simulink model "Project_2_2020a"  (R2020a)
settings: Solver=ode15s  StartTime=0.0  StopTime=10  MaxStep=0.2  RelTol=1e-2  EnableMultiTasking=on
model workspace (MAT data in the model file):
  g_density = 5
values from neighbouring files (symbols this model uses):
  Aa = 0    [execute_model_2020a.m]
  Ab = 0    [execute_model_2020a.m]
  Ac = 0    [execute_model_2020a.m]
  Ax = 0    [execute_model_2020a.m]
  Ay = 0    [execute_model_2020a.m]
  Az = 0    [execute_model_2020a.m]
  B = [24.233423136094 6.1219332628706 -6.1219332628706 -24.233423136094 -18.111489873223 18.111489873223 ... (first row only)    [execute_model_2020a.m]
  flange_len = 3    [execute_model_2020a.m]
  flange_thick = 0.8    [execute_model_2020a.m]
  flange_width = 2.25    [execute_model_2020a.m]
  hex_skew = -0.25    [execute_model_2020a.m]
  ka = 0    [execute_model_2020a.m]
  kb = 0    [execute_model_2020a.m]
  kc = 0    [execute_model_2020a.m]
  Kd = 8    [execute_model_2020a.m]
  Ki = 11.5    [execute_model_2020a.m]
  Kp = 450    [execute_model_2020a.m]
  kx = 0    [execute_model_2020a.m]
  ky = 0    [execute_model_2020a.m]
  kz = 75    [execute_model_2020a.m]
  leg_rad = 3    [execute_model_2020a.m]
  nom_length = 30    [execute_model_2020a.m]
  P = [14.574164873203 11.040422061358 -11.040422061358 -14.574164873203 -3.5337428118454 3.5337428118454 ... (first row only)    [execute_model_2020a.m]
  pa = 0    [execute_model_2020a.m]
  pb = 0    [execute_model_2020a.m]
  pc = 0    [execute_model_2020a.m]
  platform_rad = 18    [execute_model_2020a.m]
  platform_thick = 2    [execute_model_2020a.m]
  px = 0    [execute_model_2020a.m]
  py = 0    [execute_model_2020a.m]
  pz = 0    [execute_model_2020a.m]
  wa = 0    [execute_model_2020a.m]
  wb = 0    [execute_model_2020a.m]
  wc = 0    [execute_model_2020a.m]
  wx = 0    [execute_model_2020a.m]
  wy = 0    [execute_model_2020a.m]
  wz = 0    [execute_model_2020a.m]
undefined symbols (not defined in the file or in its folder): X, Y, Z
libraries: sm_stewart_platform_lib x13, sm_lib x10, nesl_utility x8, simulink x2, Parts_Lib x1, Contact_Forces_Lib x1, simulink_extras x1
(part 1 of 2)
Description:
  | Stewart Platform
  | 
  | This model shows a Stewart platform manipulator that can track a
  | parameterized reference trajectory. The shape, size, and kinematics of
  | the manipulator are highly configurable.
  | 
  | The reference trajectory is
  | specified in 6-D pose space, and an inverse kinematics module
  | converts it into one through 6-D leg position space.  A generic PID
  | controller attempts to drive the manipulator along the desired
  | trajectory.
settings Model: FPTRunName=Active  Creator=The MathWorks, Inc.  LastModifiedBy=sjain238
settings SolverCC: ZeroCrossAlgorithm=Adaptive
settings DataIOCC: LimitDataPoints=on  SaveFormat=Array  ReturnWorkspaceOutputs=off
settings OptimizationCC: ExpressionDepthLimit=2147483647  LifeSpan=inf
settings DebuggingCC: UnderspecifiedInitializationDetection=Classic  MergeDetectMultiDrivingBlocksExec=none  IgnoredZcDiagnostic=none  SolverPrmCheckMsg=warning  FcnCallInpInsideContextMsg=warning  StateNameClashWarn=warning  SFUnexpectedBacktrackingDiag=warning  SFNoUnconditionalDefaultTransitionDiag=warning  SFExecutionAtInitializationDiag=none  ArithmeticOperatorsInVariantConditions=warning
settings HardwareCC: ProdBitPerPointer=32  ProdBitPerSizeT=32  ProdBitPerPtrDiffT=32  ProdLargestAtomicFloat=None  ProdIntDivRoundTo=Undefined  ProdEndianess=Unspecified  ProdWordSize=32  ProdHWDeviceType=32-bit Generic
settings ModelReferenceCC: PropagateSignalLabelsOutOfModel=off
settings SFSimCC: SimUseLocalCustomCode=off  CustomCodeUndefinedFunction=UseInterfaceOnly
settings RTWCC: RTWUseLocalCustomCode=off
settings CodeAppCC: StateflowObjectComments=on
settings GRTTargetCC: TargetLangStandard=C89/C90 (ANSI)  CombineOutputUpdateFcns=off  GRTInterface=on
settings ConfigComp: CovMetricSettings=dw  CovSaveCumulativeToWorkspaceVar=on  CovSaveSingleToWorkspaceVar=on  CovExternalEMLEnable=off
settings SimscapeCC: SimscapeNormalizeSystem=off  SimscapeLogDataHistory=15000
settings ConfigurationSet: Description=SimMechanics 2G
settings DiagnosticsConfigSet: SimMechanicsRigidlyBoundBlock=none

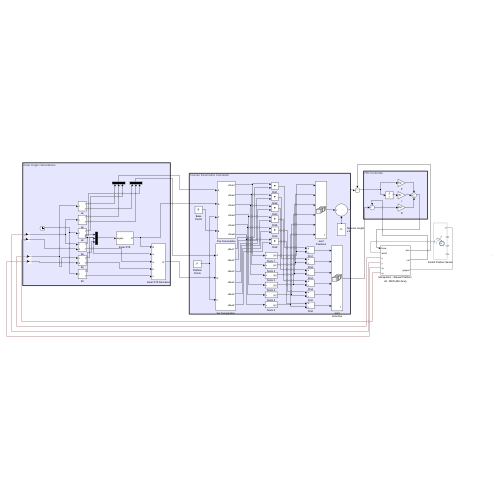
[thumbnail: Simulink's stored preview of the top-level diagram]
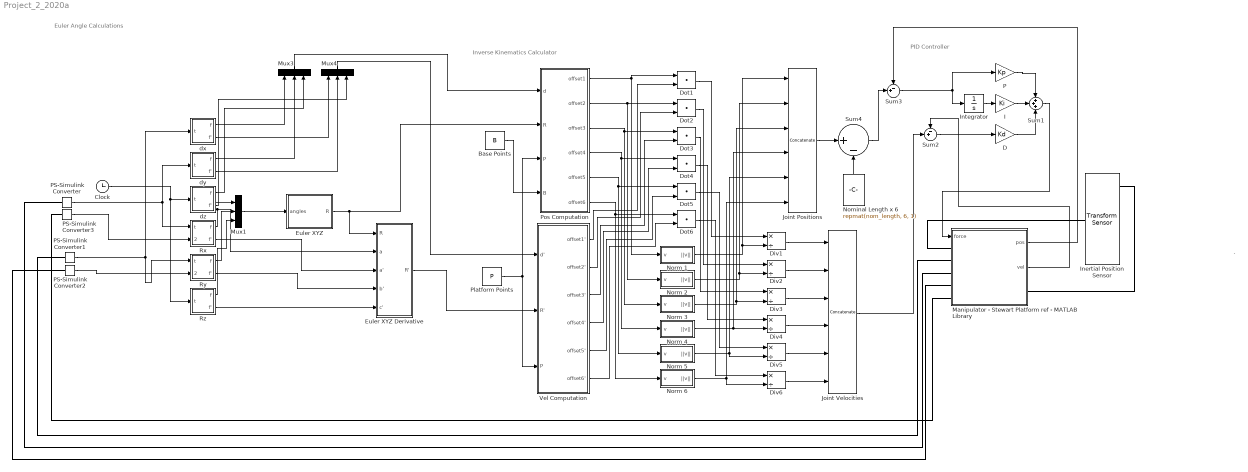
== system Project_2_2020a ==
  note: Inverse Kinematics Calculator
  note: PID Controller
  note: Euler Angle Calculations
  note: `
  Base Points : Constant  Value=B
  Clock : Clock
  D : Gain  Gain=Kd  SaturateOnIntegerOverflow=on  OutDataTypeStr=Inherit: Same as input  ParamDataTypeStr=Inherit: Same as input
  Div{1..6} (6 alike) : Product  Inputs=*/
  Dot{1..6} (6 alike) : DotProduct  OutDataTypeStr=Inherit: Inherit via internal rule
  Euler XYZ : Subsystem
  Euler XYZ Derivative : Subsystem
  I : Gain  Gain=Ki  SaturateOnIntegerOverflow=on  OutDataTypeStr=Inherit: Same as input  ParamDataTypeStr=Inherit: Same as input
  Inertial Position Sensor : sm_lib/Frames and Transforms/Transform Sensor  MeasurementFrame=World  SenseAngle=off  SenseAxis=off  SenseQ=off  SenseR=off  SenseRotationSequence=off  RotationSequence=XYX  SenseOmegaX=off  SenseOmegaY=off  SenseOmegaZ=off  SenseQDot=off  SenseRDot=off  SenseAlphaX=off  SenseAlphaY=off  SenseAlphaZ=off  SenseQDDot=off  SenseRDDot=off  SenseX=on  SenseY=on  SenseZ=on  SenseRad=off  SenseAzim=off  SenseDist=off  SenseInc=off  SenseXDot=off  SenseYDot=off  SenseZDot=off  SenseRadDot=off  SenseAzimDot=off  SenseDistDot=off  SenseIncDot=off  SenseXDDot=off  SenseYDDot=off  SenseZDDot=off  SenseRadDDot=off  SenseAzimDDot=off  SenseDistDDot=off  SenseIncDDot=off
  Integrator : Integrator  ZeroCross=off
  Joint Positions : Concatenate  NumInputs=6  Mode=Multidimensional array
  Joint Velocities : Concatenate  NumInputs=6  Mode=Multidimensional array
  Manipulator - Stewart Platform ref - MATLAB Library : Subsystem
  Mux1 : Mux  Inputs=3
  Mux3 : Mux  Inputs=3
  Mux4 : Mux  Inputs=3
  Nominal Length x 6 : Constant  Value=repmat(nom_length, 6, 1)
  Norm 1 : Subsystem
  Norm 2 : Subsystem
  Norm 3 : Subsystem
  Norm 4 : Subsystem
  Norm 5 : Subsystem
  Norm 6 : Subsystem
  P : Gain  Gain=Kp  SaturateOnIntegerOverflow=on  OutDataTypeStr=Inherit: Same as input  ParamDataTypeStr=Inherit: Same as input
  PS-Simulink Converter{,1..3} (4 alike) : nesl_utility/PS-Simulink Converter  PhysicalDomain=network_engine_domain  SubClassName=ps_output  LeftPortType=input  RightPortType=output  PseudoPeriodic=off  Frequencies=[]  VectorFormat=inherit  Unit=inherit  AffineConversion=off
  Platform Points : Constant  Value=P
  Pos Computation : Subsystem
  Rx : Subsystem  mask(Sinusoidal Trajectory){A=Aa * pi/180, w=wa, p=pa, k=ka * pi/180}
      mask prompts: A "Amplitude"; w "Frequency (deg / s)"; p "Phase (deg)"; k "Offset"
      mask help: Produces a time-varying sinusoid parameterized by amplitude, frequency, phase, and offset. Also produces the first time derivative of this function.
      mask Help:
      | A <em>Sinusoidal Trajectory</em> produces a time-varying sinusoid
      |  parameterized by amplitude, frequency, phase, and offset.  It also produces the
      |  first time derivative of this function.
      | 
      | <h3>Sinsoidal Functions</h3>
      | 
      | An arbitrary sinusoidal function of time and its first time derivative are given by
      | 
      |     f(t) = A sin (w t + p) + k
      |     f'(t) = w A cos (w t + p),
      | 
      | where <em>t</em> is time, and <em>A, w, p,</em> and <em>k</em> are scalar
      | constants.  Given time as an input signal, this block provides the f(t) and
      | f'(t) signals based on the parameters described above.
      | 
      | 
      | <h3>Parameters</h3>
      | 
      | The four parameters specify the scalar parameters described above:
      | 
      | <ul>
      | 
      | <li> <b>A</b> The <em>amplitude</em> of the sinusoid.
      | 
      | <li> <b>w</b> The <em>angular frequency</em> of the sinusoid.
      | 
      | <li> <b>p</b> The <em>phase</em> of the sinusoid.
      | 
      | <li> <b>k</b> The <em>offset</em> of the sinusoid.
      | 
      | </ul>
      | 
      | </ul>
      | 
      | <h3>Ports</h3>
      | 
      | <ul>
      | 
      | <li><b>t</b> The time function, provided as an input signal.
      | 
      | <li><b>f</b> The sinusoid f(t), as described above, as an output signal.
      | 
      | <li><b>f'</b> The sinusoid's first time derivative f'(t), as described above, as an output signal.
      | 
      | </ul>
  Ry : Subsystem  mask(Sinusoidal Trajectory){A=Ab * pi/180, w=wb, p=pb, k=kb * pi/180}
      mask prompts: A "Amplitude"; w "Frequency (deg / s)"; p "Phase (deg)"; k "Offset"
      mask help: Produces a time-varying sinusoid parameterized by amplitude, frequency, phase, and offset. Also produces the first time derivative of this function.
      mask Help:
      | A <em>Sinusoidal Trajectory</em> produces a time-varying sinusoid
      |  parameterized by amplitude, frequency, phase, and offset.  It also produces the
      |  first time derivative of this function.
      | 
      | <h3>Sinsoidal Functions</h3>
      | 
      | An arbitrary sinusoidal function of time and its first time derivative are given by
      | 
      |     f(t) = A sin (w t + p) + k
      |     f'(t) = w A cos (w t + p),
      | 
      | where <em>t</em> is time, and <em>A, w, p,</em> and <em>k</em> are scalar
      | constants.  Given time as an input signal, this block provides the f(t) and
      | f'(t) signals based on the parameters described above.
      | 
      | 
      | <h3>Parameters</h3>
      | 
      | The four parameters specify the scalar parameters described above:
      | 
      | <ul>
      | 
      | <li> <b>A</b> The <em>amplitude</em> of the sinusoid.
      | 
      | <li> <b>w</b> The <em>angular frequency</em> of the sinusoid.
      | 
      | <li> <b>p</b> The <em>phase</em> of the sinusoid.
      | 
      | <li> <b>k</b> The <em>offset</em> of the sinusoid.
      | 
      | </ul>
      | 
      | </ul>
      | 
      | <h3>Ports</h3>
      | 
      | <ul>
      | 
      | <li><b>t</b> The time function, provided as an input signal.
      | 
      | <li><b>f</b> The sinusoid f(t), as described above, as an output signal.
      | 
      | <li><b>f'</b> The sinusoid's first time derivative f'(t), as described above, as an output signal.
      | 
      | </ul>
  Rz : Subsystem  mask(Sinusoidal Trajectory){A=Ac * pi/180, w=wc, p=pc, k=kc * pi/180}
      mask prompts: A "Amplitude"; w "Frequency (deg / s)"; p "Phase (deg)"; k "Offset"
      mask help: Produces a time-varying sinusoid parameterized by amplitude, frequency, phase, and offset. Also produces the first time derivative of this function.
      mask Help:
      | A <em>Sinusoidal Trajectory</em> produces a time-varying sinusoid
      |  parameterized by amplitude, frequency, phase, and offset.  It also produces the
      |  first time derivative of this function.
      | 
      | <h3>Sinsoidal Functions</h3>
      | 
      | An arbitrary sinusoidal function of time and its first time derivative are given by
      | 
      |     f(t) = A sin (w t + p) + k
      |     f'(t) = w A cos (w t + p),
      | 
      | where <em>t</em> is time, and <em>A, w, p,</em> and <em>k</em> are scalar
      | constants.  Given time as an input signal, this block provides the f(t) and
      | f'(t) signals based on the parameters described above.
      | 
      | 
      | <h3>Parameters</h3>
      | 
      | The four parameters specify the scalar parameters described above:
      | 
      | <ul>
      | 
      | <li> <b>A</b> The <em>amplitude</em> of the sinusoid.
      | 
      | <li> <b>w</b> The <em>angular frequency</em> of the sinusoid.
      | 
      | <li> <b>p</b> The <em>phase</em> of the sinusoid.
      | 
      | <li> <b>k</b> The <em>offset</em> of the sinusoid.
      | 
      | </ul>
      | 
      | </ul>
      | 
      | <h3>Ports</h3>
      | 
      | <ul>
      | 
      | <li><b>t</b> The time function, provided as an input signal.
      | 
      | <li><b>f</b> The sinusoid f(t), as described above, as an output signal.
      | 
      | <li><b>f'</b> The sinusoid's first time derivative f'(t), as described above, as an output signal.
      | 
      | </ul>
  Sum1 : Sum  Inputs=+++  InputSameDT=on  SaturateOnIntegerOverflow=on  OutDataTypeStr=Inherit: Same as first input
  Sum2 : Sum  Inputs=-+|  InputSameDT=on  SaturateOnIntegerOverflow=on  OutDataTypeStr=Inherit: Same as first input
  Sum3 : Sum  Inputs=-+|  InputSameDT=on  SaturateOnIntegerOverflow=on  OutDataTypeStr=Inherit: Same as first input
  Sum4 : Sum  Inputs=|+-
  Vel Computation : Subsystem
  dx : Subsystem  mask(Sinusoidal Trajectory){A=Ax, w=wx, p=px, k=kx}
      mask prompts: A "Amplitude"; w "Frequency (deg / s)"; p "Phase (deg)"; k "Offset"
      mask help: Produces a time-varying sinusoid parameterized by amplitude, frequency, phase, and offset. Also produces the first time derivative of this function.
      mask Help:
      | A <em>Sinusoidal Trajectory</em> produces a time-varying sinusoid
      |  parameterized by amplitude, frequency, phase, and offset.  It also produces the
      |  first time derivative of this function.
      | 
      | <h3>Sinsoidal Functions</h3>
      | 
      | An arbitrary sinusoidal function of time and its first time derivative are given by
      | 
      |     f(t) = A sin (w t + p) + k
      |     f'(t) = w A cos (w t + p),
      | 
      | where <em>t</em> is time, and <em>A, w, p,</em> and <em>k</em> are scalar
      | constants.  Given time as an input signal, this block provides the f(t) and
      | f'(t) signals based on the parameters described above.
      | 
      | 
      | <h3>Parameters</h3>
      | 
      | The four parameters specify the scalar parameters described above:
      | 
      | <ul>
      | 
      | <li> <b>A</b> The <em>amplitude</em> of the sinusoid.
      | 
      | <li> <b>w</b> The <em>angular frequency</em> of the sinusoid.
      | 
      | <li> <b>p</b> The <em>phase</em> of the sinusoid.
      | 
      | <li> <b>k</b> The <em>offset</em> of the sinusoid.
      | 
      | </ul>
      | 
      | </ul>
      | 
      | <h3>Ports</h3>
      | 
      | <ul>
      | 
      | <li><b>t</b> The time function, provided as an input signal.
      | 
      | <li><b>f</b> The sinusoid f(t), as described above, as an output signal.
      | 
      | <li><b>f'</b> The sinusoid's first time derivative f'(t), as described above, as an output signal.
      | 
      | </ul>
  dy : Subsystem  mask(Sinusoidal Trajectory){A=Ay, w=wy, p=py, k=ky}
      mask prompts: A "Amplitude"; w "Frequency (deg / s)"; p "Phase (deg)"; k "Offset"
      mask help: Produces a time-varying sinusoid parameterized by amplitude, frequency, phase, and offset. Also produces the first time derivative of this function.
      mask Help:
      | A <em>Sinusoidal Trajectory</em> produces a time-varying sinusoid
      |  parameterized by amplitude, frequency, phase, and offset.  It also produces the
      |  first time derivative of this function.
      | 
      | <h3>Sinsoidal Functions</h3>
      | 
      | An arbitrary sinusoidal function of time and its first time derivative are given by
      | 
      |     f(t) = A sin (w t + p) + k
      |     f'(t) = w A cos (w t + p),
      | 
      | where <em>t</em> is time, and <em>A, w, p,</em> and <em>k</em> are scalar
      | constants.  Given time as an input signal, this block provides the f(t) and
      | f'(t) signals based on the parameters described above.
      | 
      | 
      | <h3>Parameters</h3>
      | 
      | The four parameters specify the scalar parameters described above:
      | 
      | <ul>
      | 
      | <li> <b>A</b> The <em>amplitude</em> of the sinusoid.
      | 
      | <li> <b>w</b> The <em>angular frequency</em> of the sinusoid.
      | 
      | <li> <b>p</b> The <em>phase</em> of the sinusoid.
      | 
      | <li> <b>k</b> The <em>offset</em> of the sinusoid.
      | 
      | </ul>
      | 
      | </ul>
      | 
      | <h3>Ports</h3>
      | 
      | <ul>
      | 
      | <li><b>t</b> The time function, provided as an input signal.
      | 
      | <li><b>f</b> The sinusoid f(t), as described above, as an output signal.
      | 
      | <li><b>f'</b> The sinusoid's first time derivative f'(t), as described above, as an output signal.
      | 
      | </ul>
  dz : Subsystem  mask(Sinusoidal Trajectory){A=Az, w=wz, p=pz, k=kz}
      mask prompts: A "Amplitude"; w "Frequency (deg / s)"; p "Phase (deg)"; k "Offset"
      mask help: Produces a time-varying sinusoid parameterized by amplitude, frequency, phase, and offset. Also produces the first time derivative of this function.
      mask Help:
      | A <em>Sinusoidal Trajectory</em> produces a time-varying sinusoid
      |  parameterized by amplitude, frequency, phase, and offset.  It also produces the
      |  first time derivative of this function.
      | 
      | <h3>Sinsoidal Functions</h3>
      | 
      | An arbitrary sinusoidal function of time and its first time derivative are given by
      | 
      |     f(t) = A sin (w t + p) + k
      |     f'(t) = w A cos (w t + p),
      | 
      | where <em>t</em> is time, and <em>A, w, p,</em> and <em>k</em> are scalar
      | constants.  Given time as an input signal, this block provides the f(t) and
      | f'(t) signals based on the parameters described above.
      | 
      | 
      | <h3>Parameters</h3>
      | 
      | The four parameters specify the scalar parameters described above:
      | 
      | <ul>
      | 
      | <li> <b>A</b> The <em>amplitude</em> of the sinusoid.
      | 
      | <li> <b>w</b> The <em>angular frequency</em> of the sinusoid.
      | 
      | <li> <b>p</b> The <em>phase</em> of the sinusoid.
      | 
      | <li> <b>k</b> The <em>offset</em> of the sinusoid.
      | 
      | </ul>
      | 
      | </ul>
      | 
      | <h3>Ports</h3>
      | 
      | <ul>
      | 
      | <li><b>t</b> The time function, provided as an input signal.
      | 
      | <li><b>f</b> The sinusoid f(t), as described above, as an output signal.
      | 
      | <li><b>f'</b> The sinusoid's first time derivative f'(t), as described above, as an output signal.
      | 
      | </ul>
  wires:
  PS-Simulink Converter3/1 -> Rx/2(Inport)
  PS-Simulink Converter2/1 -> Ry/2(Inport)
  PS-Simulink Converter1/1 -> Ry/1(t), dx/1(t)
  PS-Simulink Converter/1 -> Rx/1(t), dy/1(t)
  Mux1/1 -> Euler XYZ/1(angles)
  Rz/2(f') -> Euler XYZ Derivative/5(c')
  Ry/2(f') -> Euler XYZ Derivative/4(b')
  Rx/2(f') -> Euler XYZ Derivative/3(a')
  Rz/1(f) -> Mux1/3
  Ry/1(f) -> Mux1/2
  Clock/1 -> Rz/1(t), dz/1(t)
  Rx/1(f) -> Mux1/1, Euler XYZ Derivative/2(a)
  dz/2(f') -> Mux4/3
  dy/2(f') -> Mux4/2
  dx/2(f') -> Mux4/1
  dz/1(f) -> Mux3/3
  dy/1(f) -> Mux3/2
  dx/1(f) -> Mux3/1
  Sum1/1 -> Manipulator - Stewart Platform ref - MATLAB Library/1(force)
  D/1 -> Sum1/3
  Joint Velocities/1 -> Sum2/2
  Manipulator - Stewart Platform ref - MATLAB Library/2(vel) -> Sum2/1
  Sum4/1 -> Sum3/2
  Manipulator - Stewart Platform ref - MATLAB Library/1(pos) -> Sum3/1
  Sum3/1 -> P/1, Integrator/1
  I/1 -> Sum1/2
  P/1 -> Sum1/1
  Integrator/1 -> I/1
  Sum2/1 -> D/1
  Dot1/1 -> Div1/1
  Vel Computation/1(offset1') -> Dot1/2
  Euler XYZ Derivative/1(R') -> Vel Computation/2(R')
  Div5/1 -> Joint Velocities/5
  Div4/1 -> Joint Velocities/4
  Div3/1 -> Joint Velocities/3
  Div6/1 -> Joint Velocities/6
  Div2/1 -> Joint Velocities/2
  Div1/1 -> Joint Velocities/1
  Dot3/1 -> Div3/1
  Dot4/1 -> Div4/1
  Dot5/1 -> Div5/1
  Dot6/1 -> Div6/1
  Dot2/1 -> Div2/1
  Mux4/1 -> Vel Computation/1(d')
  Vel Computation/6(offset6') -> Dot6/2
  Vel Computation/5(offset5') -> Dot5/2
  Vel Computation/2(offset2') -> Dot2/2
  Vel Computation/4(offset4') -> Dot4/2
  Vel Computation/3(offset3') -> Dot3/2
  Norm 5/1(||v||) -> Joint Positions/5, Div5/2
  Norm 4/1(||v||) -> Joint Positions/4, Div4/2
  Norm 3/1(||v||) -> Joint Positions/3, Div3/2
  Norm 2/1(||v||) -> Joint Positions/2, Div2/2
  Norm 6/1(||v||) -> Joint Positions/6, Div6/2
  Norm 1/1(||v||) -> Joint Positions/1, Div1/2
  Pos Computation/6(offset6) -> Norm 6/1(v), Dot6/1
  Pos Computation/5(offset5) -> Norm 5/1(v), Dot5/1
  Pos Computation/1(offset1) -> Norm 1/1(v), Dot1/1
  Pos Computation/2(offset2) -> Norm 2/1(v), Dot2/1
  Pos Computation/3(offset3) -> Norm 3/1(v), Dot3/1
  Pos Computation/4(offset4) -> Norm 4/1(v), Dot4/1
  Platform Points/1 -> Pos Computation/3(P), Vel Computation/3(P)
  Base Points/1 -> Pos Computation/4(B)
  Euler XYZ/1(R) -> Pos Computation/2(R), Euler XYZ Derivative/1(R)
  Mux3/1 -> Pos Computation/1(d)
  Nominal Length x 6/1 -> Sum4/2
  Joint Positions/1 -> Sum4/1
  connections:
  Manipulator - Stewart Platform ref - MATLAB Library/LConn3 -- PS-Simulink Converter/LConn1
  Manipulator - Stewart Platform ref - MATLAB Library/LConn4 -- PS-Simulink Converter2/LConn1
  Manipulator - Stewart Platform ref - MATLAB Library/LConn5 -- PS-Simulink Converter3/LConn1
  Manipulator - Stewart Platform ref - MATLAB Library/LConn2 -- PS-Simulink Converter1/LConn1
  Manipulator - Stewart Platform ref - MATLAB Library/RConn1 -- Inertial Position Sensor/RConn1
  Manipulator - Stewart Platform ref - MATLAB Library/LConn1 -- Inertial Position Sensor/LConn1

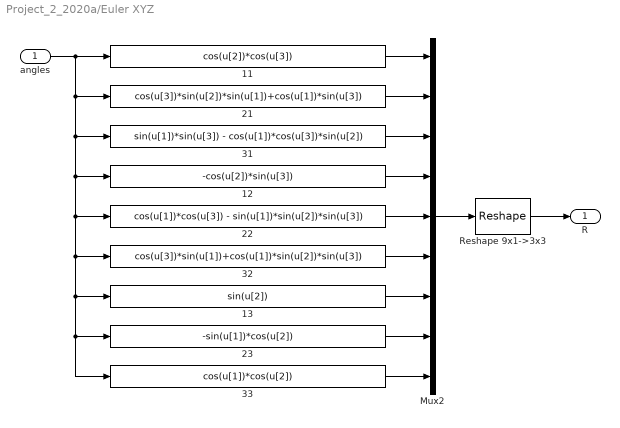
== system Project_2_2020a/Euler XYZ ==
  angles : Inport
  11 : Fcn  Expr=cos(u[2])*cos(u[3])
  12 : Fcn  Expr=-cos(u[2])*sin(u[3])
  13 : Fcn  Expr=sin(u[2])
  21 : Fcn  Expr=cos(u[3])*sin(u[2])*sin(u[1])+cos(u[1])*sin(u[3])
  22 : Fcn  Expr=cos(u[1])*cos(u[3]) - sin(u[1])*sin(u[2])*sin(u[3])
  23 : Fcn  Expr=-sin(u[1])*cos(u[2])
  31 : Fcn  Expr=sin(u[1])*sin(u[3]) - cos(u[1])*cos(u[3])*sin(u[2])
  32 : Fcn  Expr=cos(u[3])*sin(u[1])+cos(u[1])*sin(u[2])*sin(u[3])
  33 : Fcn  Expr=cos(u[1])*cos(u[2])
  Mux2 : Mux  Inputs=9
  Reshape 9x1->3x3 : Reshape  OutputDimensionality=Customize  OutputDimensions=[3,3]
  R : Outport  VectorParamsAs1DForOutWhenUnconnected=off
  wires:
  angles/1 -> 23/1, 33/1, 13/1, 32/1, 22/1, 12/1, 31/1, 21/1, 11/1
  33/1 -> Mux2/9
  23/1 -> Mux2/8
  13/1 -> Mux2/7
  32/1 -> Mux2/6
  22/1 -> Mux2/5
  12/1 -> Mux2/4
  31/1 -> Mux2/3
  21/1 -> Mux2/2
  11/1 -> Mux2/1
  Mux2/1 -> Reshape 9x1->3x3/1
  Reshape 9x1->3x3/1 -> R/1

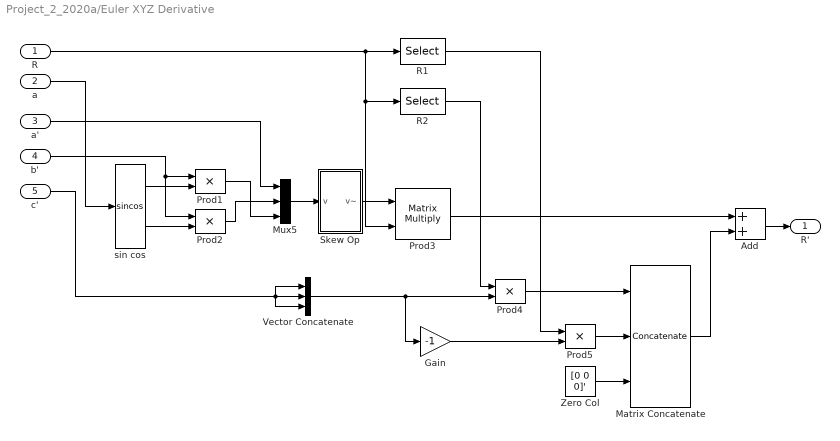
== system Project_2_2020a/Euler XYZ Derivative ==
  R : Inport
  a : Inport  Port=2
  a' : Inport  Port=3
  b' : Inport  Port=4
  c' : Inport  Port=5
  Add : Sum
  Gain : Gain  Gain=-1
  Matrix Concatenate : Concatenate  NumInputs=3  Mode=Multidimensional array  ConcatenateDimension=2
  Mux5 : Mux  Inputs=3
  Prod{1..2,4..5} (4 alike) : Product  RndMeth=Zero
  Prod3 : Product  Multiplication=Matrix(*)  RndMeth=Zero
  R1 : Selector  NumberOfDimensions=2  InputPortWidth=3  IndexOptions=Select all,Index vector (dialog)  Indices=[1 3],1  OutputSizes=1,1
  R2 : Selector  NumberOfDimensions=2  InputPortWidth=3  IndexOptions=Select all,Index vector (dialog)  Indices=[1 3],2  OutputSizes=1,1
  Skew Op : Subsystem
  Vector Concatenate : Concatenate  NumInputs=3  Mode=Multidimensional array
  Zero Col : Constant  Value=[0 0 0]'
  sin cos : Trigonometry  Operator=sincos
  R' : Outport  VectorParamsAs1DForOutWhenUnconnected=off
  wires:
  a/1 -> sin cos/1
  sin cos/1 -> Prod1/2
  sin cos/2 -> Prod2/2
  b'/1 -> Prod2/1, Prod1/1
  a'/1 -> Mux5/1
  Prod2/1 -> Mux5/2
  Prod1/1 -> Mux5/3
  Mux5/1 -> Skew Op/1(v)
  Vector Concatenate/1 -> Prod4/2, Gain/1
  R2/1 -> Prod4/1
  Gain/1 -> Prod5/2
  Zero Col/1 -> Matrix Concatenate/3
  Prod5/1 -> Matrix Concatenate/2
  Prod4/1 -> Matrix Concatenate/1
  R1/1 -> Prod5/1
  Prod3/1 -> Add/1
  Matrix Concatenate/1 -> Add/2
  Add/1 -> R'/1
  R/1 -> R1/1, Prod3/2, R2/1
  Skew Op/1(v~) -> Prod3/1
  c'/1 -> Vector Concatenate/2, Vector Concatenate/1, Vector Concatenate/3

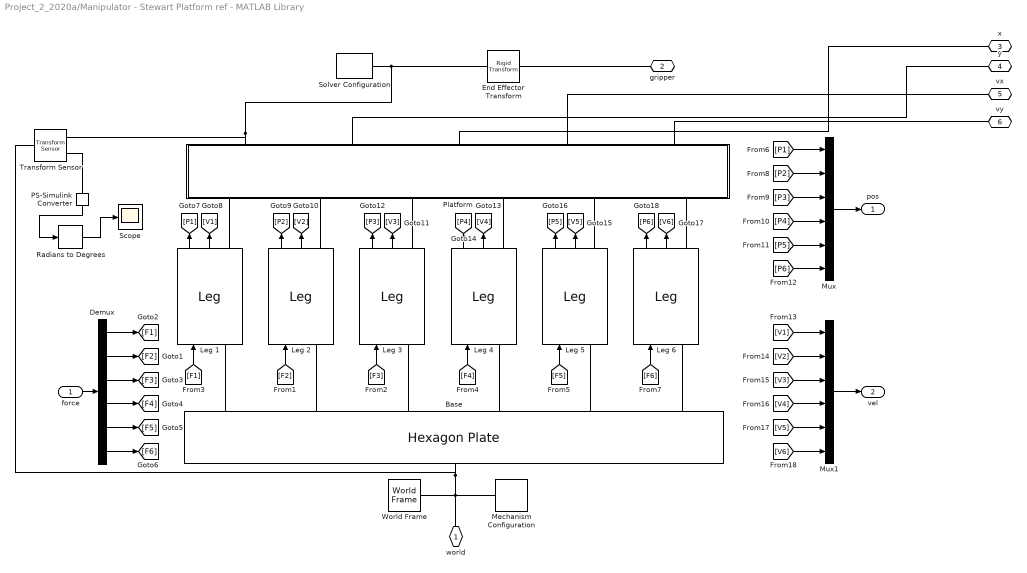
== system Project_2_2020a/Manipulator - Stewart Platform ref - MATLAB Library ==
  force : Inport
  Base : sm_stewart_platform_lib/Hexagon Plate  kind=base  hex_rad=base_rad  hex_thick=base_thick  hex_skew=hex_skew  flange_sep=2 * leg_rad * cos(pi/6) - flange_thick  flange_len=flange_len  flange_width=flange_width  flange_thick=flange_thick  diffuse=[0.4 0.3 0.2 0.5]  specular=[0 0 0]  shininess=10
  Demux : Demux  Outputs=6
  End Effector Transform : sm_lib/Frames and Transforms/Rigid Transform  TranslationMethod=StandardAxis  TranslationStandardOffset=platform_thick / 2  TranslationLengthUnit=cm  TranslationStandardAxis=+Z  TranslationCartesianOffset=[0 0 0]  TranslationROffset=0  TranslationROffsetUnits=m  TranslationZOffset=0  TranslationZOffsetUnits=m  TranslationThetaOffset=0  TranslationThetaOffsetUnits=deg  RotationMethod=StandardAxis  RotationAngleUnits=rad  RotationStandardAxis=+Z  RotationAngle=pi/3  RotationArbitraryAxis=[0 0 1]  FollAlignAxisA=+X  BaseAlignAxisA=+Y  FollAlignAxisB=+Y  BaseAlignAxisB=+Z  RotationSequenceAxes=FollowerAxes  RotationSequence=XYX  RotationSequenceAngles=[0 0 0]  RotationSequenceAnglesUnits=deg  RotationMatrix=[1 0 0; 0 1 0; 0 0 1]  Quaternion=[1 0 0 0]
  Leg {1..6} (6 alike) : sm_stewart_platform_lib/Leg  upper_leg_len=upper_leg_len  lower_leg_len=lower_leg_len  rad=leg_rad  collar_thick=collar_thick  flange_len=flange_len  flange_width=flange_width  flange_thick=flange_thick  asm_offset=asm_offset
  Mechanism Configuration : sm_lib/Utilities/Mechanism Configuration  UniformGravity=Constant  GravityVector=[0 0 -9.81]  GravityUnits=m/s^2  LinearizationDelta=0.001  JointModeTransitionNonlinearIterations=2
  Mux : Mux  Inputs=6
  Mux1 : Mux  Inputs=6
  PS-Simulink Converter : nesl_utility/PS-Simulink Converter  PhysicalDomain=network_engine_domain  SubClassName=ps_output  LeftPortType=input  RightPortType=output  PseudoPeriodic=off  Frequencies=[]  VectorFormat=inherit  Unit=inherit  AffineConversion=off
  Platform : Subsystem  AncestorBlock=sm_stewart_platform_lib/Hexagon Plate  mask(Hexagon Plate){kind=platform, hex_rad=platform_rad, hex_thick=platform_thick, hex_skew=hex_skew, flange_sep=2 * leg_rad * cos(pi/6) - flange_thick, flange_len=flange_len, flange_width=flange_width, flange_thick=flange_thick, diffuse=[.7 .7 .3 0.75], specular=[.7 .7 .3 0.75], shininess=90}
      mask prompts: hex_rad "Hexagon Radius (cm)"; hex_thick "Hexagon Thickness (cm)"; hex_skew "Hexagon Skew"; flange_sep "Flange Separation (cm)"; flange_len "Flange Length (cm)"; flange_width "Flange Width (cm)"; flange_thick "Flange Thickness (cm)"; diffuse "Diffuse (rgba)"; specular "Specular (rgba)"
      mask help:
      | Models a rigid body formed by attaching six couplings to the corners of a skewed hexagon.
      |
      | There are two hexagon plates in a Stewart platform manipulator: one forming the grounded base, and the other forming the moveable platform.  Six legs connect the corresponding couplings of these two plates.  Both plates are modeled with this block.
      mask init:
      | % Set up a value equal to 0 or 1 based on whether
      | % this is the base or platform, respectively.  This value
      | % is used in the computations of certain variables and
      | % transforms that differ for the two types of hexagon plates.
      | if (kind == 1)
      |     kind_val = 0;  % Value for base
      | else
      |     kind_val = 1;  % Value for platform
      | end
      mask Help:
      | A <em>Hexagon Plate</em> models a rigid body formed by attaching six couplings to the corners of a skewed hexagon.
      | 
      | There are two hexagon plates in a Stewart platform manipulator: one forming the grounded base, and the other forming the moveable platform.  Six legs connect the corresponding couplings of these two plates.  Both plates are modeled with this block.
      | 
      | <h3>Skewed Hexagons</h3>
      | 
      | The main part of a hexagon plate is a </em>skewed hexagon</em>.  This is short hexagonal prism.  The cross section is based on a regular hexagon, but with the vertices perturbed according to the skew factor, a real value in the range (-0.5, +0.5).
      | 
      | The vertices of a skewed hexagon always lie on a circle centered at the origin. The ith vertex (i = 1, 2, ..., 6) is located at the intersection of the ray at angle theta_i with this circle, where theta_i is given by
      | 
      | theta_i = [ i - 1 + (-1)^(i - 1) s ] * pi/3  radians,
      | 
      | where s is the skew factor.  A skew factor of zero produces vertices around the circle at angles 0, pi/3, 2/3 pi, pi, 4/3 pi, 5/3 pi.  In other words, the vertices form a regular hexagon.
      | 
      | As the skew factor increase in magnitude, the hexagon vertices are shifted so that the shape becomes more and more triangular, as pairs of vertices approach each another.  Three of the sides of the hexagon grow longer as the other three grow shorter.  Regardless of the skew factor, the skewed hexagon exhibits 3-fold symmetry.  It exhibits 6-fold symmetry for a zero skew factor only.  When the skew factor is +/- 1, pairs of vertices overlap and the cross section becomes an equilateral triangle; this configuration is degenerate and not allowed.
      | 
      | A skew factor of -s produces the same shape as a skew factor of +s, except that the three side that lengthen under a skew factor of +s shrink under a skew factor of -s, and vice versa.  For a hexagonal plate, this affects the way couplings are placed on the hexagon.  If the skew factor is positive, the couplings are placed along the long sides of the hexagon; if the skew factor is negative, the couplings are placed along the short sides.
      | 
      | <h3>Geometry</h3>
      | 
      | The <em>Geom</em> tab parameters specify the geometry of the hexagon plate.
      | 
      | <ul>
      | 
      | <li> <b>Kind</b> An enumerated parameter with possible values of <em>base</em> or <em>platform</em>.  This affects some computations that are slightly different for the two types of hexagon plates in a Stewart platform.  The differences stem from two reasons.  First, the couplings appear on the top side of the base plate but on the underside of the platform plate.  Second, the couplings indices on the platform plate are offset by one (modulo 6) relative to the coupling indices on the base plate.  This causes the legs of the platform to lean in directions tangential to the edges of the base and platform plates, which adds stability to the manipulator.
      | 
      | <li> <b>Hexagon Radius</b> The radius of the circle on which the vertices of the hexagonal cross section lie.
      | 
      | <li> <b>Hexagon Thickness</b> The thickness (length) of the hexagonal prism forming the main part of the hexagon plate.
      | 
      | <li> <b>Hexagon Skew</b> The skew factor of the hexagonal cross section, in the range (-0.5, +0.5).  See <em>Skewed Hexagons</em> above for details.
      | 
      | </ul>
      | 
      | <h3>Flanges</h3>
      | 
      | The <em>Flanges</em> tab parameters specify the geometry of the flanges of the six couplings of the hexagonal plate.
      | 
      | <ul>
      | 
      | <li> <b>Flange Separation</b> The flange separation of the couplings of the hexagon plate.  See <em>Coupling</em> block for details.
      | 
      | <li> <b>Flange Length</b> The length of the coupling flanges. See <em>Coupling</em> block for details.
      | 
      | <li> <b>Flange Width</b> The width of the coupling flanges. See <em>Coupling</em> block for details.
      | 
      | <li> <b>Flange Thickness</b> The thickness of the coupling flanges. See <em>Coupling</em> block for details.
      | 
      | </ul>
      | 
      | <h3>Visualization</h3>
      | 
      | The <em>Graphics</em> tab parameters specify the visualization aspects of the hexagon plate.  The skewed hexagon and all six couplings share the same visual properties.
      | 
      | <ul>
      | 
      | <li> <b>Diffuse</b> The diffuse color of the hexagon plate.  This is an RGB 3-vector or an RGBA 4-vector with all components in the range [0, 1].
      | 
      | <li> <b>Specular</b> The specular color of the hexagon plate.  This is an RGB 3-vector or an RGBA 4-vector with all components in the range [0, 1].
      | 
      | <li> <b>Shininess</b> The shininess of the hexagon plate.  This is a scalar value in the range [0, 128].
      | 
      | </ul>
      | 
      | 
      | <h3>Ports</h3>
      | 
      | <ul>
      | 
      | <li> <b>ref</b> Reference frame of the hexagon plate.  The origin of this frame is located at the center of the skewed hexagon prism.  For a base plate, this frame is typically attached to ground or a supporting body.  For the platform plate, this frame is used to define an attachment point for a payload or end effector.
      | 
      | <li> <b>leg1, ..., leg6</b> Attachment frames for the six legs of the Stewart platform.  Each leg is attached to one of these six frames through one of its crosspieces.  When all six legs are connected to both hexagon plates in this manner, the result is a kinematically valid Stewart platform manipulator.
      | 
      | </ul>
      mask TypeOptions kind: base | platform
      mask Display:
      | image('sm_stewart_platform_hexagonplate.png')
      | color('white')
      | port_label('LConn', 1, 'ref')
      | port_label('RConn', 1, 'leg1')
      | port_label('RConn', 2, 'leg2')
      | port_label('RConn', 3, 'leg3')
      | port_label('RConn', 4, 'leg4')
      | port_label('RConn', 5, 'leg5')
      | port_label('RConn', 6, 'leg6')
  Radians to Degrees : simulink_extras/Transformations/Radians to Degrees
  Scope : Scope
  Solver Configuration : nesl_utility/Solver Configuration  PhysicalDomain=network_engine_domain  SubClassName=solver  LeftPortType=input  RightPortType=generic  Tones=[]  Harmonics=[]  SimulateNoise=off  Profile=off  UseLocalSampling=off  EnableSwitchedLinearOptims=on  FrequencyDomain=off  UseCCode=off  RelTol=0.001  AbsTol=0.001  MinStep=1e-09  ToWorkspace=off  RevertToSquareIcSolve=off  NumHomotopyIterations=100  PhasorMode=off  PhasorModeNumHarmonics=1  ConsistencySolver=NEWTON_FTOL  IndexReductionMethod=DerivativeReplacement  DoDC=off  ResidualTolerance=1e-9  ConsistencyTolSource=GLOBAL  ConsistencyAbsTol=0.001  ConsistencyRelTol=0.001  ConsistencyTolFactor=0.001  UseLocalSolver=off  LocalSolverChoice=NE_BACKWARD_EULER_ADVANCER  ResolveIndetEquations=on  FunctionEvalNumThread=1  LocalSolverSampleTime=.001  DoFixedCost=off  MaxNonlinIter=3  MaxModeIter=2  ComputeImpulses=off  ImpulseIterations=2  LinearAlgebra=Sparse  LinearAlgebraNumThread=0  EquationFormulation=NE_TIME_EF  DelaysMemoryBudget=1024  AutomaticFiltering=on  FilteringTimeConstant=0.001  PartitionStorageMethod=AS_NEEDED  PartitionMemoryBudget=1024  PartitionMethod=FAST
  Transform Sensor : sm_lib/Frames and Transforms/Transform Sensor  MeasurementFrame=World  SenseAngle=on  SenseAxis=off  SenseQ=off  SenseR=off  SenseRotationSequence=off  RotationSequence=XYX  SenseOmegaX=off  SenseOmegaY=off  SenseOmegaZ=off  SenseQDot=off  SenseRDot=off  SenseAlphaX=off  SenseAlphaY=off  SenseAlphaZ=off  SenseQDDot=off  SenseRDDot=off  SenseX=off  SenseY=off  SenseZ=off  SenseRad=off  SenseAzim=off  SenseDist=off  SenseInc=off  SenseXDot=off  SenseYDot=off  SenseZDot=off  SenseRadDot=off  SenseAzimDot=off  SenseDistDot=off  SenseIncDot=off  SenseXDDot=off  SenseYDDot=off  SenseZDDot=off  SenseRadDDot=off  SenseAzimDDot=off  SenseDistDDot=off  SenseIncDDot=off
  World Frame : sm_lib/Frames and Transforms/World Frame
  world : PMIOPort  Side=Left
  gripper : PMIOPort  Port=2  Side=Right
  x : PMIOPort  Port=3  Side=Left
  y : PMIOPort  Port=4  Side=Left
  vx : PMIOPort  Port=5  Side=Left
  vy : PMIOPort  Port=6  Side=Left
  pos : Outport  VectorParamsAs1DForOutWhenUnconnected=off
  vel : Outport  Port=2  VectorParamsAs1DForOutWhenUnconnected=off
  wires:
  Demux/1 -> [F1]
  Demux/2 -> [F2]
  Demux/3 -> [F3]
  Demux/4 -> [F4]
  Demux/5 -> [F5]
  Demux/6 -> [F6]
  [F1] -> Leg 1/1
  [F2] -> Leg 2/1
  [F3] -> Leg 3/1
  [F4] -> Leg 4/1
  [F5] -> Leg 5/1
  [F6] -> Leg 6/1
  force/1 -> Demux/1
  Leg 1/1 -> [P1]
  Leg 1/2 -> [V1]
  Leg 2/1 -> [P2]
  Leg 2/2 -> [V2]
  Leg 3/1 -> [P3]
  Leg 3/2 -> [V3]
  Leg 4/1 -> [P4]
  Leg 4/2 -> [V4]
  Leg 5/1 -> [P5]
  Leg 5/2 -> [V5]
  Leg 6/1 -> [P6]
  Leg 6/2 -> [V6]
  Mux/1 -> pos/1
  [P1] -> Mux/1
  [P2] -> Mux/2
  [P3] -> Mux/3
  [P4] -> Mux/4
  [P5] -> Mux/5
  [P6] -> Mux/6
  [V1] -> Mux1/1
  [V2] -> Mux1/2
  [V3] -> Mux1/3
  [V4] -> Mux1/4
  [V5] -> Mux1/5
  [V6] -> Mux1/6
  Mux1/1 -> vel/1
  Radians to Degrees/1 -> Scope/1
  PS-Simulink Converter/1 -> Radians to Degrees/1
  connections:
  Platform/LConn1 -- End Effector Transform/LConn1 -- Solver Configuration/RConn1 -- Transform Sensor/RConn1
  Mechanism Configuration/RConn1 -- world/RConn1 -- Transform Sensor/LConn1 -- Base/LConn1 -- World Frame/RConn1
  Base/RConn6 -- Leg 6/LConn1
  Base/RConn5 -- Leg 5/LConn1
  Base/RConn2 -- Leg 2/LConn1
  Base/RConn1 -- Leg 1/LConn1
  Base/RConn3 -- Leg 3/LConn1
  Base/RConn4 -- Leg 4/LConn1
  Leg 1/RConn1 -- Platform/RConn1
  Leg 2/RConn1 -- Platform/RConn2
  Leg 5/RConn1 -- Platform/RConn5
  Leg 6/RConn1 -- Platform/RConn6
  Leg 3/RConn1 -- Platform/RConn3
  Leg 4/RConn1 -- Platform/RConn4
  Platform/LConn3 -- x/RConn1
  Platform/LConn2 -- y/RConn1
  Platform/LConn4 -- vx/RConn1
  Platform/LConn5 -- vy/RConn1
  Transform Sensor/RConn2 -- PS-Simulink Converter/LConn1
  gripper/RConn1 -- End Effector Transform/RConn1

== system Project_2_2020a/Norm 1 ==
  v : Inport
  Dot Product : DotProduct  OutDataTypeStr=Inherit: Inherit via internal rule
  Sqrt : Sqrt  SaturateOnIntegerOverflow=on
  ||v|| : Outport  VectorParamsAs1DForOutWhenUnconnected=off
  wires:
  Dot Product/1 -> Sqrt/1
  Sqrt/1 -> ||v||/1
  v/1 -> Dot Product/1, Dot Product/2

== system Project_2_2020a/Norm 2 ==
  v : Inport
  Dot Product : DotProduct  OutDataTypeStr=Inherit: Inherit via internal rule
  Sqrt : Sqrt  SaturateOnIntegerOverflow=on
  ||v|| : Outport  VectorParamsAs1DForOutWhenUnconnected=off
  wires:
  Dot Product/1 -> Sqrt/1
  Sqrt/1 -> ||v||/1
  v/1 -> Dot Product/1, Dot Product/2

== system Project_2_2020a/Norm 3 ==
  v : Inport
  Dot Product : DotProduct  OutDataTypeStr=Inherit: Inherit via internal rule
  Sqrt : Sqrt  SaturateOnIntegerOverflow=on
  ||v|| : Outport  VectorParamsAs1DForOutWhenUnconnected=off
  wires:
  Dot Product/1 -> Sqrt/1
  Sqrt/1 -> ||v||/1
  v/1 -> Dot Product/1, Dot Product/2

== system Project_2_2020a/Norm 4 ==
  v : Inport
  Dot Product : DotProduct  OutDataTypeStr=Inherit: Inherit via internal rule
  Sqrt : Sqrt  SaturateOnIntegerOverflow=on
  ||v|| : Outport  VectorParamsAs1DForOutWhenUnconnected=off
  wires:
  Dot Product/1 -> Sqrt/1
  Sqrt/1 -> ||v||/1
  v/1 -> Dot Product/1, Dot Product/2

== system Project_2_2020a/Norm 5 ==
  v : Inport
  Dot Product : DotProduct  OutDataTypeStr=Inherit: Inherit via internal rule
  Sqrt : Sqrt  SaturateOnIntegerOverflow=on
  ||v|| : Outport  VectorParamsAs1DForOutWhenUnconnected=off
  wires:
  Dot Product/1 -> Sqrt/1
  Sqrt/1 -> ||v||/1
  v/1 -> Dot Product/1, Dot Product/2

== system Project_2_2020a/Norm 6 ==
  v : Inport
  Dot Product : DotProduct  OutDataTypeStr=Inherit: Inherit via internal rule
  Sqrt : Sqrt  SaturateOnIntegerOverflow=on
  ||v|| : Outport  VectorParamsAs1DForOutWhenUnconnected=off
  wires:
  Dot Product/1 -> Sqrt/1
  Sqrt/1 -> ||v||/1
  v/1 -> Dot Product/1, Dot Product/2

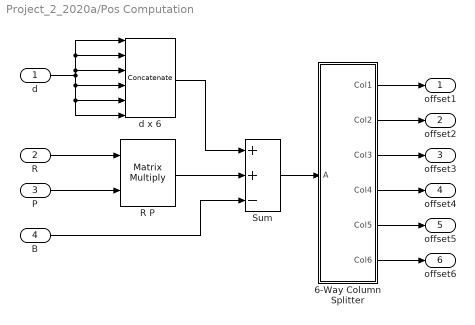
== system Project_2_2020a/Pos Computation ==
  d : Inport
  R : Inport  Port=2
  P : Inport  Port=3
  B : Inport  Port=4
  6-Way Column Splitter : Subsystem
  R P : Product  Multiplication=Matrix(*)  RndMeth=Zero
  Sum : Sum  Inputs=++-
  d x 6 : Concatenate  NumInputs=6  Mode=Multidimensional array  ConcatenateDimension=2
  offset1 : Outport  VectorParamsAs1DForOutWhenUnconnected=off
  offset2 : Outport  Port=2  VectorParamsAs1DForOutWhenUnconnected=off
  offset3 : Outport  Port=3  VectorParamsAs1DForOutWhenUnconnected=off
  offset4 : Outport  Port=4  VectorParamsAs1DForOutWhenUnconnected=off
  offset5 : Outport  Port=5  VectorParamsAs1DForOutWhenUnconnected=off
  offset6 : Outport  Port=6  VectorParamsAs1DForOutWhenUnconnected=off
  wires:
  d/1 -> d x 6/3, d x 6/2, d x 6/1, d x 6/4, d x 6/5, d x 6/6
  Sum/1 -> 6-Way Column Splitter/1(A)
  6-Way Column Splitter/1(Col1) -> offset1/1
  R/1 -> R P/1
  6-Way Column Splitter/2(Col2) -> offset2/1
  6-Way Column Splitter/3(Col3) -> offset3/1
  6-Way Column Splitter/4(Col4) -> offset4/1
  6-Way Column Splitter/5(Col5) -> offset5/1
  6-Way Column Splitter/6(Col6) -> offset6/1
  d x 6/1 -> Sum/1
  R P/1 -> Sum/2
  P/1 -> R P/2
  B/1 -> Sum/3

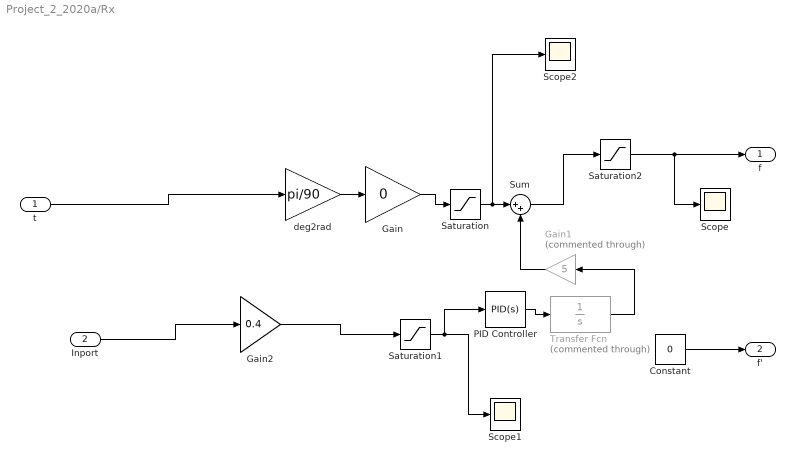
== system Project_2_2020a/Rx ==
  t : Inport
  Inport : Inport  Port=2
  Constant : Constant  Value=0
  Gain : Gain  Gain=0
  Gain1 : Gain  Commented=through  Gain=5
  Gain2 : Gain  Gain=0.4
  PID Controller : simulink/Continuous/PID Controller  Controller=PID  Form=Parallel  TimeDomain=Continuous-time  UseExternalTs=off  SampleTime=-1  IntegratorMethod=Forward Euler  ControllerParametersSource=internal  P=15  I=8  D=2  N=100  UseFilter=on  TunerSelectOption=Transfer Function Based (PID Tuner App)  InitialConditionSource=internal  InitialConditionForIntegrator=0  InitialConditionForFilter=0  DifferentiatorICPrevScaledInput=0  ExternalReset=none  TrackingMode=off  Kt=1  LimitOutput=off  UpperSaturationLimit=inf  LowerSaturationLimit=-inf  LinearizeAsGain=on  AntiWindupMode=none  Kb=1  POutMin=[]  POutMax=[]  IOutMin=[]  IOutMax=[]  DOutMin=[]  DOutMax=[]  NOutMin=[]  NOutMax=[]  SumOutMin=[]  SumOutMax=[]  SaturationOutMin=[]  SaturationOutMax=[]  PParamMin=[]  PParamMax=[]  IParamMin=[]  IParamMax=[]  DParamMin=[]  DParamMax=[]  NParamMin=[]  NParamMax=[]  KbParamMin=[]  KbParamMax=[]  KtParamMin=[]  KtParamMax=[]  KbOutMin=[]  KbOutMax=[]  KtOutMin=[]  KtOutMax=[]  IntegratorOutMin=[]  IntegratorOutMax=[]  FilterOutMin=[]  FilterOutMax=[]  SumI1OutMin=[]  SumI1OutMax=[]  SumI2OutMin=[]  SumI2OutMax=[]  SumI3OutMin=[]  SumI3OutMax=[]  SumI4OutMin=[]  SumI4OutMax=[]  SumDOutMin=[]  SumDOutMax=[]  DifferentiatorOutMin=[]  DifferentiatorOutMax=[]  FilterDiffOutCoefMin=[]  FilterDiffOutCoefMax=[]  ReciprocalOutMin=[]  ReciprocalOutMax=[]  SumDenOutMin=[]  SumDenOutMax=[]  SumNumOutMin=[]  SumNumOutMax=[]  DivideOutMin=[]  DivideOutMax=[]  UdiffTsProdOutMin=[]  UdiffTsProdOutMax=[]  NTsProdOutMin=[]  NTsProdOutMax=[]  UintegralTsProdOutMin=[]  UintegralTsProdOutMax=[]  UngainTsProdOutMin=[]  UngainTsProdOutMax=[]  IntegratorContinuousStateAttributes=''  IntegratorStateMustResolveToSignalObject=off  IntegratorRTWStateStorageClass=Auto  FilterContinuousStateAttributes=''  FilterStateMustResolveToSignalObject=off  FilterRTWStateStorageClass=Auto  ParallelPVariant=InternalParameters  IdealPVariant=Disabled  IVariant=InternalParameters  DVariant=InternalParameters  IntegratorVariant=Continuous  SatVariant=Disabled  AWVariant=Passthrough  PCopyVariant=Disabled  TRVariant=Disabled  FdbkBlocksVariant=Forward  IdealPFdbkVariant=Disabled  SatFdbkVariant=Disabled  DerivativeFilterVariant=ContFilter  NVariant=InternalParameters  NCopyVariant=Disabled  FilterICVariant=InternalICsFilter  IntegratorICVariant=InternalICs  ExternalResetVariant=Disabled  TRSumVariant=Passthrough  SumFdbkVariant=Disabled  SumVariant=Sum_PID  TsampFilterVariant=InternalTs  TsampNgainVariant=Passthrough  TsampIntegralVariant=Passthrough
  Saturation : Saturate  UpperLimit=0.2  LowerLimit=-0.2
  Saturation1 : Saturate  UpperLimit=0.4  LowerLimit=-0.4
  Saturation2 : Saturate  UpperLimit=0.15  LowerLimit=-0.15
  Scope : Scope
  Scope1 : Scope
  Scope2 : Scope
  Sum : Sum  Inputs=|++
  Transfer Fcn : TransferFcn  Commented=through  Denominator=[1 0]
  deg2rad : Gain  Gain=pi/90
  f : Outport  VectorParamsAs1DForOutWhenUnconnected=off
  f' : Outport  Port=2  VectorParamsAs1DForOutWhenUnconnected=off
  wires:
  deg2rad/1 -> Gain/1
  Saturation1/1 -> PID Controller/1, Scope1/1
  Gain2/1 -> Saturation1/1
  Inport/1 -> Gain2/1
  Gain/1 -> Saturation/1
  t/1 -> deg2rad/1
  Transfer Fcn/1 -> Gain1/1
  Saturation/1 -> Scope2/1, Sum/1
  Sum/1 -> Saturation2/1
  Gain1/1 -> Sum/2
  Saturation2/1 -> Scope/1, f/1
  Constant/1 -> f'/1
  PID Controller/1 -> Transfer Fcn/1

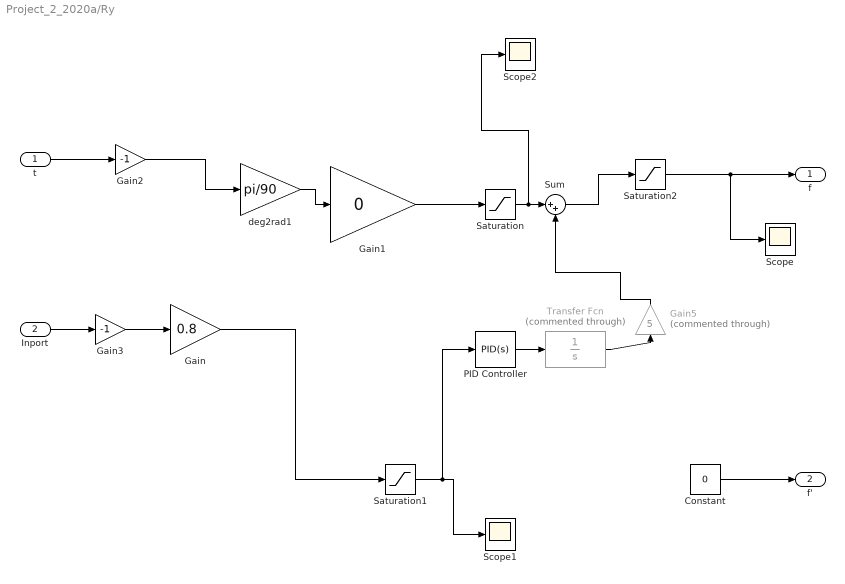
== system Project_2_2020a/Ry ==
  t : Inport
  Inport : Inport  Port=2
  Constant : Constant  Value=0
  Gain : Gain  Gain=0.8
  Gain1 : Gain  Gain=0
  Gain2 : Gain  Gain=-1
  Gain3 : Gain  Gain=-1
  Gain5 : Gain  Commented=through  Gain=5
  PID Controller : simulink/Continuous/PID Controller  Controller=PID  Form=Parallel  TimeDomain=Continuous-time  UseExternalTs=off  SampleTime=-1  IntegratorMethod=Forward Euler  ControllerParametersSource=internal  P=15  I=8  D=2  N=100  UseFilter=on  TunerSelectOption=Transfer Function Based (PID Tuner App)  InitialConditionSource=internal  InitialConditionForIntegrator=0  InitialConditionForFilter=0  DifferentiatorICPrevScaledInput=0  ExternalReset=none  TrackingMode=off  Kt=1  LimitOutput=off  UpperSaturationLimit=inf  LowerSaturationLimit=-inf  LinearizeAsGain=on  AntiWindupMode=none  Kb=1  POutMin=[]  POutMax=[]  IOutMin=[]  IOutMax=[]  DOutMin=[]  DOutMax=[]  NOutMin=[]  NOutMax=[]  SumOutMin=[]  SumOutMax=[]  SaturationOutMin=[]  SaturationOutMax=[]  PParamMin=[]  PParamMax=[]  IParamMin=[]  IParamMax=[]  DParamMin=[]  DParamMax=[]  NParamMin=[]  NParamMax=[]  KbParamMin=[]  KbParamMax=[]  KtParamMin=[]  KtParamMax=[]  KbOutMin=[]  KbOutMax=[]  KtOutMin=[]  KtOutMax=[]  IntegratorOutMin=[]  IntegratorOutMax=[]  FilterOutMin=[]  FilterOutMax=[]  SumI1OutMin=[]  SumI1OutMax=[]  SumI2OutMin=[]  SumI2OutMax=[]  SumI3OutMin=[]  SumI3OutMax=[]  SumI4OutMin=[]  SumI4OutMax=[]  SumDOutMin=[]  SumDOutMax=[]  DifferentiatorOutMin=[]  DifferentiatorOutMax=[]  FilterDiffOutCoefMin=[]  FilterDiffOutCoefMax=[]  ReciprocalOutMin=[]  ReciprocalOutMax=[]  SumDenOutMin=[]  SumDenOutMax=[]  SumNumOutMin=[]  SumNumOutMax=[]  DivideOutMin=[]  DivideOutMax=[]  UdiffTsProdOutMin=[]  UdiffTsProdOutMax=[]  NTsProdOutMin=[]  NTsProdOutMax=[]  UintegralTsProdOutMin=[]  UintegralTsProdOutMax=[]  UngainTsProdOutMin=[]  UngainTsProdOutMax=[]  IntegratorContinuousStateAttributes=''  IntegratorStateMustResolveToSignalObject=off  IntegratorRTWStateStorageClass=Auto  FilterContinuousStateAttributes=''  FilterStateMustResolveToSignalObject=off  FilterRTWStateStorageClass=Auto  ParallelPVariant=InternalParameters  IdealPVariant=Disabled  IVariant=InternalParameters  DVariant=InternalParameters  IntegratorVariant=Continuous  SatVariant=Disabled  AWVariant=Passthrough  PCopyVariant=Disabled  TRVariant=Disabled  FdbkBlocksVariant=Forward  IdealPFdbkVariant=Disabled  SatFdbkVariant=Disabled  DerivativeFilterVariant=ContFilter  NVariant=InternalParameters  NCopyVariant=Disabled  FilterICVariant=InternalICsFilter  IntegratorICVariant=InternalICs  ExternalResetVariant=Disabled  TRSumVariant=Passthrough  SumFdbkVariant=Disabled  SumVariant=Sum_PID  TsampFilterVariant=InternalTs  TsampNgainVariant=Passthrough  TsampIntegralVariant=Passthrough
  Saturation : Saturate  UpperLimit=0.2  LowerLimit=-0.2
  Saturation1 : Saturate  UpperLimit=0.4  LowerLimit=-0.4
  Saturation2 : Saturate  UpperLimit=0.15  LowerLimit=-0.15
  Scope : Scope
  Scope1 : Scope
  Scope2 : Scope
  Sum : Sum  Inputs=|++
  Transfer Fcn : TransferFcn  Commented=through  Denominator=[1 0]
  deg2rad1 : Gain  Gain=pi/90
  f : Outport  VectorParamsAs1DForOutWhenUnconnected=off
  f' : Outport  Port=2  VectorParamsAs1DForOutWhenUnconnected=off
  wires:
  Inport/1 -> Gain3/1
  Gain/1 -> Saturation1/1
  Gain1/1 -> Saturation/1
  t/1 -> Gain2/1
  deg2rad1/1 -> Gain1/1
  Saturation1/1 -> PID Controller/1, Scope1/1
  Gain2/1 -> deg2rad1/1
  Gain3/1 -> Gain/1
  Sum/1 -> Saturation2/1
  Saturation/1 -> Scope2/1, Sum/1
  Transfer Fcn/1 -> Gain5/1
  Constant/1 -> f'/1
  Gain5/1 -> Sum/2
  Saturation2/1 -> Scope/1, f/1
  PID Controller/1 -> Transfer Fcn/1

== system Project_2_2020a/Rz ==
  t : Inport
  Add : Sum  Inputs=|++
  Add2 : Sum  Inputs=++|
  amp1 : Gain  Gain=A
  amp2 : Gain  Gain=w*A*pi/180
  deg2rad : Gain  Gain=pi/180
  freq : Gain  Gain=w
  offset : Constant  Value=k  VectorParams1D=off
  phase : Constant  Value=p  VectorParams1D=off
  sin cos : Trigonometry  Operator=sincos
  f : Outport  VectorParamsAs1DForOutWhenUnconnected=off
  f' : Outport  Port=2  VectorParamsAs1DForOutWhenUnconnected=off
  wires:
  t/1 -> freq/1
  Add/1 -> deg2rad/1
  phase/1 -> Add/2
  amp2/1 -> f'/1
  Add2/1 -> f/1
  offset/1 -> Add2/1
  sin cos/1 -> amp1/1
  sin cos/2 -> amp2/1
  amp1/1 -> Add2/2
  freq/1 -> Add/1
  deg2rad/1 -> sin cos/1

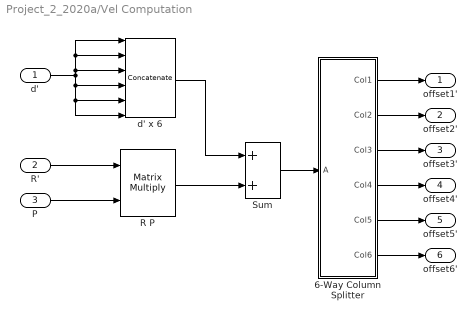
== system Project_2_2020a/Vel Computation ==
  d' : Inport
  R' : Inport  Port=2
  P : Inport  Port=3
  6-Way Column Splitter : Subsystem
  R P : Product  Multiplication=Matrix(*)  RndMeth=Zero
  Sum : Sum
  d' x 6 : Concatenate  NumInputs=6  Mode=Multidimensional array  ConcatenateDimension=2
  offset1' : Outport  VectorParamsAs1DForOutWhenUnconnected=off
  offset2' : Outport  Port=2  VectorParamsAs1DForOutWhenUnconnected=off
  offset3' : Outport  Port=3  VectorParamsAs1DForOutWhenUnconnected=off
  offset4' : Outport  Port=4  VectorParamsAs1DForOutWhenUnconnected=off
  offset5' : Outport  Port=5  VectorParamsAs1DForOutWhenUnconnected=off
  offset6' : Outport  Port=6  VectorParamsAs1DForOutWhenUnconnected=off
  wires:
  d'/1 -> d' x 6/3, d' x 6/2, d' x 6/1, d' x 6/4, d' x 6/5, d' x 6/6
  Sum/1 -> 6-Way Column Splitter/1(A)
  6-Way Column Splitter/1(Col1) -> offset1'/1
  R'/1 -> R P/1
  6-Way Column Splitter/2(Col2) -> offset2'/1
  6-Way Column Splitter/3(Col3) -> offset3'/1
  6-Way Column Splitter/4(Col4) -> offset4'/1
  6-Way Column Splitter/5(Col5) -> offset5'/1
  6-Way Column Splitter/6(Col6) -> offset6'/1
  d' x 6/1 -> Sum/1
  R P/1 -> Sum/2
  P/1 -> R P/2

== system Project_2_2020a/dx ==
  t : Inport
  Constant : Constant  Value=0
  Gain : Gain  Gain=0
  Gain1 : Gain  Gain=10
  Saturation : Saturate
  Scope : Scope
  amp2 : Gain  Gain=w*A*pi/180
  f : Outport  VectorParamsAs1DForOutWhenUnconnected=off
  f' : Outport  Port=2  VectorParamsAs1DForOutWhenUnconnected=off
  wires:
  amp2/1 -> f'/1
  t/1 -> Gain/1
  Gain/1 -> Gain1/1
  Saturation/1 -> Scope/1, f/1
  Constant/1 -> amp2/1
  Gain1/1 -> Saturation/1
